simulink model "Tarea_5"  (R2021a)
settings: Solver=VariableStepAuto  StartTime=0.0  StopTime=100  RelTol=1e-3
libraries: mpclib x2
settings Model: Creator=Seb  LastModifiedBy=Seb

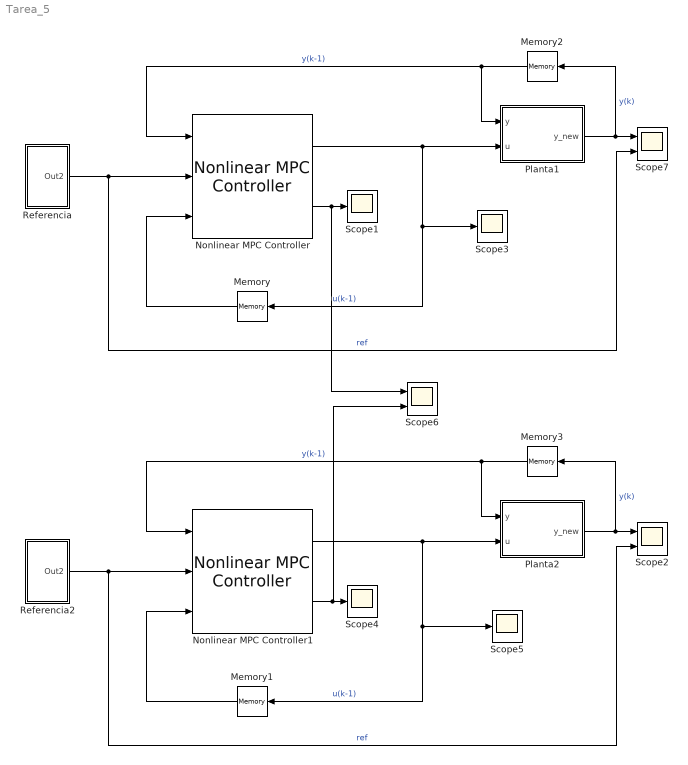
== system Tarea_5 ==
  Memory{,1..3} (4 alike) : Memory
  Nonlinear MPC Controller : mpclib/Nonlinear MPC Controller  SCDEnableBlockLinearizationSpecification=on  nlmpcobj=Controlador  UseObjectTs=on  UseMEX=off  md_enabled=off  mvtarget_enabled=off  param_enabled=off  cost_enabled=on  mvseq_enabled=off  stateseq_enabled=off  ovseq_enabled=off  slack_enabled=off  status_enabled=off  ov_min=off  ov_max=off  mv_min=off  mv_max=off  mvrate_min=off  mvrate_max=off  state_min=off  state_max=off  ov_weight=off  mv_weight=off  mvrate_weight=off  ecr_weight=off  nlp_initialize=off
  Nonlinear MPC Controller1 : mpclib/Nonlinear MPC Controller  SCDEnableBlockLinearizationSpecification=on  nlmpcobj=Controlador  UseObjectTs=on  UseMEX=off  md_enabled=off  mvtarget_enabled=off  param_enabled=off  cost_enabled=on  mvseq_enabled=off  stateseq_enabled=off  ovseq_enabled=off  slack_enabled=off  status_enabled=off  ov_min=off  ov_max=off  mv_min=off  mv_max=off  mvrate_min=off  mvrate_max=off  state_min=off  state_max=off  ov_weight=off  mv_weight=off  mvrate_weight=off  ecr_weight=off  nlp_initialize=off
  Planta1 : MATLAB Function  TreatAsAtomicUnit=on
  Planta2 : MATLAB Function  TreatAsAtomicUnit=on
  Referencia : Subsystem
  Referencia2 : Subsystem
  Scope{1,3..5} (4 alike) : Scope
  Scope2 : Scope  NumInputPorts=2
  Scope6 : Scope  NumInputPorts=2
  Scope7 : Scope  NumInputPorts=2
  wires:
  Nonlinear MPC Controller/1 -> Memory/1, Scope3/1, Planta1/2(u)  "u(k-1)"
  Referencia/1(Out2) -> Scope7/2, Nonlinear MPC Controller/2  "ref"
  Nonlinear MPC Controller/2 -> Scope6/1, Scope1/1
  Memory/1 -> Nonlinear MPC Controller/3
  Planta1/1(y_new) -> Scope7/1, Memory2/1  "y(k)"
  Memory2/1 -> Planta1/1(y), Nonlinear MPC Controller/1  "y(k-1)"
  Memory3/1 -> Nonlinear MPC Controller1/1, Planta2/1(y)  "y(k-1)"
  Planta2/1(y_new) -> Scope2/1, Memory3/1  "y(k)"
  Memory1/1 -> Nonlinear MPC Controller1/3
  Nonlinear MPC Controller1/2 -> Scope6/2, Scope4/1
  Referencia2/1(Out2) -> Scope2/2, Nonlinear MPC Controller1/2  "ref"
  Nonlinear MPC Controller1/1 -> Planta2/2(u), Memory1/1, Scope5/1  "u(k-1)"

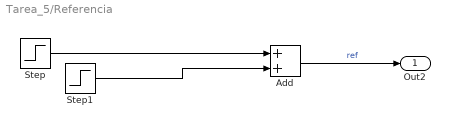
== system Tarea_5/Referencia ==
  Add : Sum
  Step : Step  Time=0  After=10.5  SampleTime=0
  Step1 : Step  Time=30  SampleTime=0
  Out2 : Outport
  wires:
  Step/1 -> Add/1
  Step1/1 -> Add/2
  Add/1 -> Out2/1  "ref"

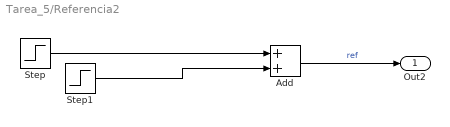
== system Tarea_5/Referencia2 ==
  Add : Sum
  Step : Step  Time=0  After=10.5  SampleTime=0
  Step1 : Step  Time=30  After=-1  SampleTime=0
  Out2 : Outport
  wires:
  Add/1 -> Out2/1  "ref"
  Step1/1 -> Add/2
  Step/1 -> Add/1

== matlab function Tarea_5/Planta2 ==
  data: y input; u input; y_new output
function y_new = Planta(y, u)
y_new = 0.8*y + 1.2 + 50*u -250*u^2;
end

== matlab function Tarea_5/Planta1 ==
  data: y input; u input; y_new output
function y_new = Planta(y, u)
y_new = 0.8*y + 1.2 + 50*u -250*u^2;
end
